simulink model "pv_control"  (R2023a)
settings: Solver=FixedStepDiscrete  StartTime=0.0  StopTime=Inf  FixedStep=Ts  RelTol=1e-3  EnableMultiTasking=on
undefined symbols (not defined in the file): dendp, denPQ, DiscIntNeverNeededParam, Down, Emax, fff, GPTRIP1SEL, GPTRIP2SEL, k, Kic, Kiv, Kpc, Kpv, L, l, m, n, numdp, numPQ, Ts, TZ1, TZ2, Up, Vdc, w
libraries: memblks x14, simulink x13, c2802xlib x12, slpidlib x9, c2837xDlib x7, spsdq0toabcLib x2, spsabctodq0Lib x2, dspswit3 x2, eeGeneralControl x1, idelinklib_common x1, spsPowerdq0InstantaneousLib x1, simulink_extras x1
(part 8 of 8)

== matlab function pv_control/PWM/MATLAB Function ==
  data: y output; Vpv input; iref output; Ipv input; Control input; d input; perr input; ierr input
function [y,iref] = P_and_O(Vpv, Ipv,Control, d,   perr, ierr)
    persistent Vold Pold iref_old Ipv_old n;
    
    if isempty(Vold) % Initialize Vold, Pold, and iref_old with isempty
        Vold = single(0);
        Pold = single(0);
        iref_old =single(0);
        Ipv_old=single(0);
        n=single(0);
    end
    
        while n<10000
        n=n+1;
        end
    dP=single(0);
    if Control==0
        Pold=Vold*Ipv_old;
        P = Vpv * Ipv;
        dP = P - Pold;
        dVpv = Vpv - Vold;
        dI = Ipv - Ipv_old;
        
            if dP > perr
                if dI > ierr
                    iref = iref_old + d; % Change iref directly inside the if loop
                else
                    iref = iref_old - d;
                end
            else
                if dI > ierr
                    iref = iref_old - d; % Change iref directly inside the if loop
                else
                    iref = iref_old + d;
                end
            end
            Vold = Vpv;
              Pold = P;
             iref_old = iref;
              Ipv_old=Ipv;
               n=single(0);
    else
        iref_old=single(0);
        iref=single(25);
        n=single(0);
    end
    y=dP;
end

== matlab function pv_control/PWM/MATLAB Function2 ==
  data: u input; y output
function y = fcn(u)
persistent x;
if isempty(x)
    x=single(0);
end
while u==1  
 x=x+single(0.25);
 y=x
 if x>=single(8)
    x=single(0);
end
end
if u==0
    x=single(0);
end

y = x;
